simulink model "Lab6"  (R2022b)
settings: Solver=FixedStepDiscrete  StartTime=0.0  StopTime=10.0  FixedStep=0.005  RelTol=1e-3
undefined symbols (not defined in the file): K_gain
settings Model: Creator=LOQ  LastModifiedBy=LOQ
settings OptimizationCC: DefaultParameterBehavior=Inlined  UseDivisionForNetSlopeComputation=on  GainParamInheritBuiltInType=on  UseFloatMulNetSlope=on  InlineInvariantSignals=on  ReuseModelBlockBuffer=on  PassReuseOutputArgsAs=Individual arguments  ZeroExternalMemoryAtStartup=off  ZeroInternalMemoryAtStartup=off  NoFixptDivByZeroProtection=on  EfficientFloat2IntCast=on  LifeSpan=1  OptimizeBlockOrder=speed  DifferentSizesBufferReuse=on  EfficientTunableParamExpr=on
settings DebuggingCC: ParameterTunabilityLossMsg=error
settings HardwareCC: ProdBitPerPointer=32  ProdBitPerSizeT=32  ProdBitPerPtrDiffT=32  ProdLargestAtomicInteger=Long  ProdLargestAtomicFloat=Double  ProdWordSize=32  ProdLongLongMode=on  ProdHWDeviceType=ARM Compatible->ARM Cortex-M
settings SFSimCC: MATLABDynamicMemAlloc=off
settings RTWCC: Description=Embedded Coder  SystemTargetFile=ert.tlc  GenCodeOnly=on  TemplateMakefile=ert_default_tmf  GenerateReport=on  GPUComputeCapability=5.0
settings CodeAppCC: ForceParamTrailComments=on  IgnoreCustomStorageClasses=off  OperatorAnnotations=on  SimulinkDataObjDesc=on  SFDataObjDesc=on  CustomSymbolStrGlobalVar=rt$N$M  CustomSymbolStrType=$N$M  CustomSymbolStrFcn=$N$M$F  CustomSymbolStrMacro=$N$M  InsertBlockDesc=on
settings ERTTargetCC: TargetLangStandard=C99 (ISO)  GenerateSampleERTMain=on  IncludeMdlTerminateFcn=off  CombineSignalStateStructs=on  SupportAbsoluteTime=off  SupportComplex=off  SupportContinuousTime=on  InlinedParameterPlacement=NonHierarchical  ERTCustomFileTemplate=example_file_process.tlc  ERTFilePackagingFormat=CompactWithDataFile
settings ConfigComp: CovBoundaryAbsTol=1.0e-5

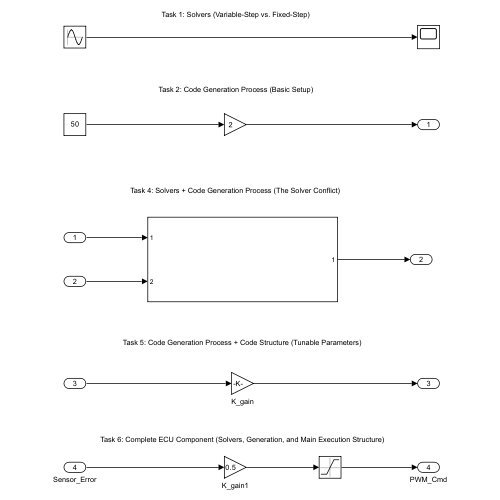
[thumbnail: Simulink's stored preview of the top-level diagram]
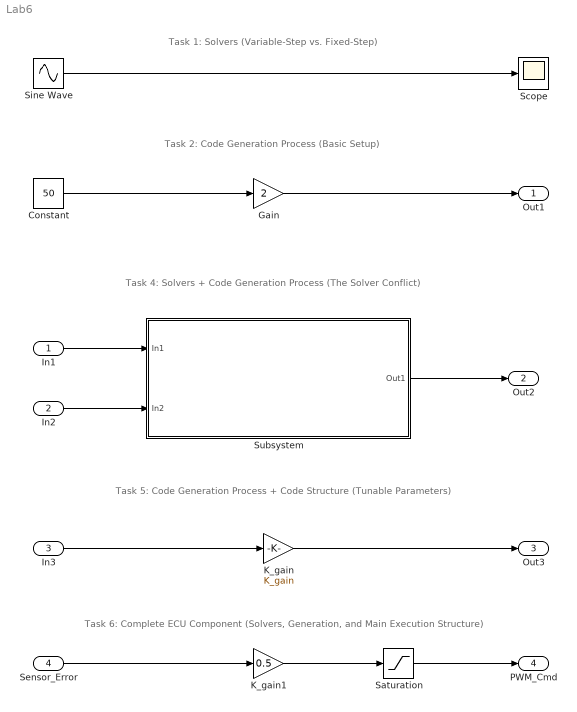
== system Lab6 ==
  note: Task 6: Complete ECU Component (Solvers, Generation, and Main Execution Structure)
  note: Task 5: Code Generation Process + Code Structure (Tunable Parameters)
  note: Task 4: Solvers + Code Generation Process (The Solver Conflict)
  note: Task 2: Code Generation Process (Basic Setup)
  note: Task 1: Solvers (Variable-Step vs. Fixed-Step)
  In1 : Inport
  In2 : Inport  Port=2
  In3 : Inport  Port=3
  Sensor_Error : Inport  Port=4
  Constant : Constant  Value=50
  Gain : Gain  Gain=2
  K_gain : Gain  Gain=K_gain
  K_gain1 : Gain  Gain=0.5
  Saturation : Saturate  UpperLimit=100  LowerLimit=0
  Scope : Scope
  Sine Wave : Sin  Amplitude=10  Frequency=5  SampleTime=0
  Subsystem : Subsystem
  Out1 : Outport
  Out2 : Outport  Port=2
  Out3 : Outport  Port=3
  PWM_Cmd : Outport  Port=4
  wires:
  Sine Wave/1 -> Scope/1
  Constant/1 -> Gain/1
  Gain/1 -> Out1/1
  In1/1 -> Subsystem/1(In1)
  In2/1 -> Subsystem/2(In2)
  Subsystem/1(Out1) -> Out2/1
  K_gain/1 -> Out3/1
  In3/1 -> K_gain/1
  K_gain1/1 -> Saturation/1
  Sensor_Error/1 -> K_gain1/1
  Saturation/1 -> PWM_Cmd/1

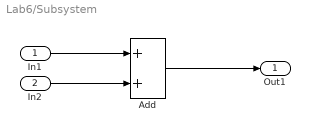
== system Lab6/Subsystem ==
  In1 : Inport
  In2 : Inport  Port=2
  Add : Sum
  Out1 : Outport
  wires:
  In1/1 -> Add/1
  In2/1 -> Add/2
  Add/1 -> Out1/1
